simulink model "exp5"  (R2023a)
settings: Solver=VariableStepAuto  StartTime=0.0  StopTime=50  RelTol=1e-3
settings Model: Creator=USER  LastModifiedBy=USER

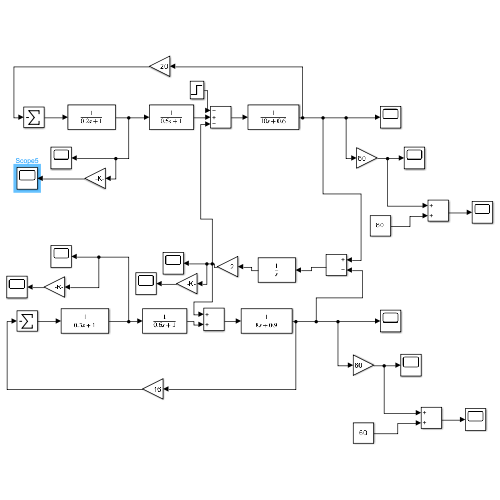
[thumbnail: Simulink's stored preview of the top-level diagram]
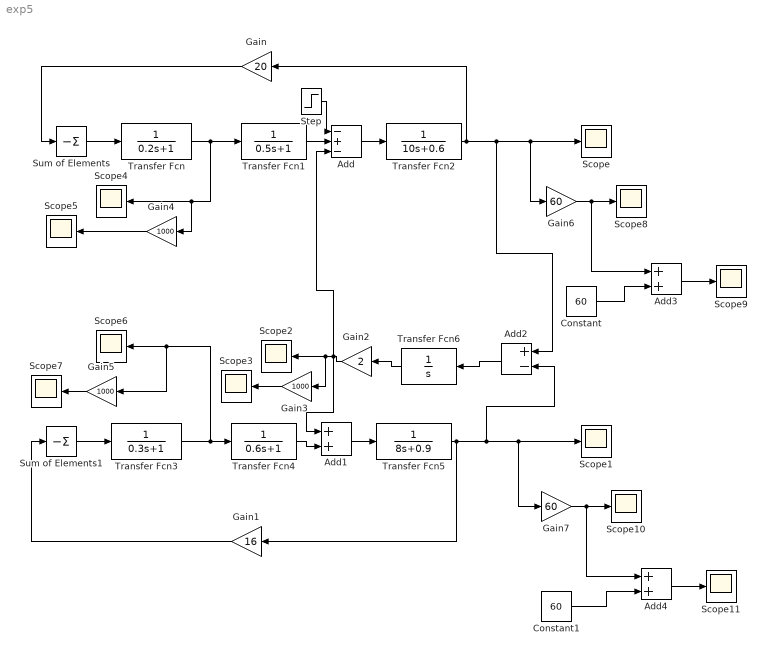
== system exp5 ==
  Add : Sum  Inputs=-+-
  Add1 : Sum
  Add2 : Sum  Inputs=+-
  Add3 : Sum
  Add4 : Sum
  Constant : Constant  Value=60
  Constant1 : Constant  Value=60
  Gain : Gain  Gain=20
  Gain1 : Gain  Gain=16
  Gain2 : Gain  Gain=2
  Gain3 : Gain  Gain=1000
  Gain4 : Gain  Gain=1000
  Gain5 : Gain  Gain=1000
  Gain6 : Gain  Gain=60
  Gain7 : Gain  Gain=60
  Scope{,1..11} (12 alike) : Scope
  Step : Step  Before=0.1875  After=0.1875  SampleTime=0
  Sum of Elements : Sum  Inputs=-
  Sum of Elements1 : Sum  Inputs=-
  Transfer Fcn : TransferFcn  Denominator=[0.2 1]
  Transfer Fcn1 : TransferFcn  Denominator=[0.5 1]
  Transfer Fcn2 : TransferFcn  Denominator=[10 0.6]
  Transfer Fcn3 : TransferFcn  Denominator=[0.3 1]
  Transfer Fcn4 : TransferFcn  Denominator=[0.6 1]
  Transfer Fcn5 : TransferFcn  Denominator=[8 0.9]
  Transfer Fcn6 : TransferFcn  Denominator=[1 0]
  wires:
  Transfer Fcn/1 -> Gain4/1, Scope4/1, Transfer Fcn1/1
  Add/1 -> Transfer Fcn2/1
  Transfer Fcn2/1 -> Gain/1, Add2/1, Gain6/1, Scope/1
  Transfer Fcn1/1 -> Add/2
  Step/1 -> Add/1
  Transfer Fcn3/1 -> Gain5/1, Scope6/1, Transfer Fcn4/1
  Add1/1 -> Transfer Fcn5/1
  Transfer Fcn4/1 -> Add1/2
  Add2/1 -> Transfer Fcn6/1
  Transfer Fcn6/1 -> Gain2/1
  Gain2/1 -> Add/3, Add1/1, Gain3/1, Scope2/1
  Gain3/1 -> Scope3/1
  Sum of Elements/1 -> Transfer Fcn/1
  Gain/1 -> Sum of Elements/1
  Gain4/1 -> Scope5/1
  Gain1/1 -> Sum of Elements1/1
  Sum of Elements1/1 -> Transfer Fcn3/1
  Gain5/1 -> Scope7/1
  Gain6/1 -> Add3/1, Scope8/1
  Constant/1 -> Add3/2
  Add3/1 -> Scope9/1
  Transfer Fcn5/1 -> Gain1/1, Add2/2, Gain7/1, Scope1/1
  Gain7/1 -> Add4/1, Scope10/1
  Constant1/1 -> Add4/2
  Add4/1 -> Scope11/1
